simulink model "FlightControllers"  (R2021a)
settings: Solver=ode4  StartTime=0.0  StopTime=200  FixedStep=0.01  RelTol=1e-3
undefined symbols (not defined in the file): g, U0
libraries: aerolibasang x1
settings Model: Creator=User01  LastModifiedBy=User01

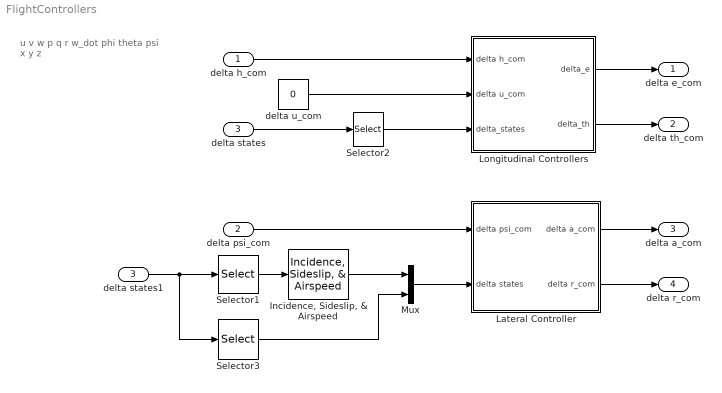
== system FlightControllers ==
  note: u
      | v
      | w
      |
      | p
      | q
      | r
      |
      | w_dot
      |
      | phi
      | theta
      | psi
      |
      | x
      | y
      | z
  delta h_com : Inport
  delta psi_com : Inport  Port=2
  delta states : Inport  Port=3
  "Incidence, Sideslip, & Airspeed" : aerolibasang/Incidence, Sideslip, & Airspeed
  Lateral Controller : Subsystem
  Longitudinal Controllers : Subsystem
  Mux : Mux  Inputs=2
  Selector1 : Selector  InputPortWidth=13  IndexOptions=Index vector (dialog)  Indices=[1:3]  OutputSizes=1
  Selector2 : Selector  InputPortWidth=13  IndexOptions=Index vector (dialog)  Indices=[1 3 5 9 13]  OutputSizes=1
  Selector3 : Selector  InputPortWidth=13  IndexOptions=Index vector (dialog)  Indices=[4 6 8 10]  OutputSizes=1
  delta states1 : InportShadow  Port=3
  delta u_com : Constant  Value=0
  delta e_com : Outport
  delta th_com : Outport  Port=2
  delta a_com : Outport  Port=3
  delta r_com : Outport  Port=4
  wires:
  Longitudinal Controllers/1(delta_e) -> delta e_com/1
  Longitudinal Controllers/2(delta_th) -> delta th_com/1
  Selector2/1 -> Longitudinal Controllers/3(delta_states)
  delta h_com/1 -> Longitudinal Controllers/1(delta h_com)
  delta states/1 -> Selector2/1
  delta u_com/1 -> Longitudinal Controllers/2(delta u_com)
  Lateral Controller/1(delta a_com) -> delta a_com/1
  Lateral Controller/2(delta r_com) -> delta r_com/1
  delta psi_com/1 -> Lateral Controller/1(delta psi_com)
  delta states1/1 -> Selector3/1, Selector1/1
  Selector1/1 -> "Incidence, Sideslip, & Airspeed"/1
  "Incidence, Sideslip, & Airspeed"/2 -> Mux/1
  Mux/1 -> Lateral Controller/2(delta states)
  Selector3/1 -> Mux/2

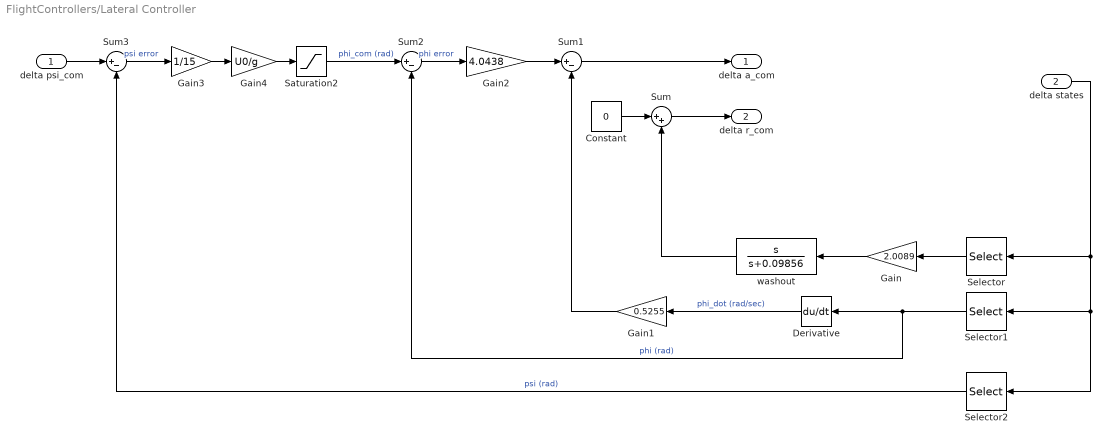
== system FlightControllers/Lateral Controller ==
  delta psi_com : Inport
  delta states : Inport  Port=2
  Constant : Constant  Value=0
  Derivative : Derivative
  Gain : Gain  Gain=2.0089
  Gain1 : Gain  Gain=0.5255
  Gain2 : Gain  Gain=4.0438
  Gain3 : Gain  Gain=1/15
  Gain4 : Gain  Gain=U0/g
  Saturation2 : Saturate  UpperLimit=30*pi/180  LowerLimit=-30*pi/180
  Selector : Selector  InputPortWidth=5  IndexOptions=Index vector (dialog)  Indices=3  OutputSizes=1
  Selector1 : Selector  InputPortWidth=5  IndexOptions=Index vector (dialog)  Indices=4  OutputSizes=1
  Selector2 : Selector  InputPortWidth=5  IndexOptions=Index vector (dialog)  Indices=5  OutputSizes=1
  Sum : Sum  Inputs=|++
  Sum1 : Sum  Inputs=|+-
  Sum2 : Sum  Inputs=|+-
  Sum3 : Sum  Inputs=|+-
  washout : TransferFcn  Numerator=[1 0]  Denominator=[1 0.09856]
  delta a_com : Outport
  delta r_com : Outport  Port=2
  wires:
  Derivative/1 -> Gain1/1  "phi_dot (rad/sec)"
  delta states/1 -> Selector2/1, Selector1/1, Selector/1
  Sum/1 -> delta r_com/1
  Sum3/1 -> Gain3/1  "psi error"
  Constant/1 -> Sum/1
  washout/1 -> Sum/2
  Gain2/1 -> Sum1/1
  Gain/1 -> washout/1
  Selector/1 -> Gain/1
  Saturation2/1 -> Sum2/1  "phi_com (rad)"
  Sum2/1 -> Gain2/1  "phi error"
  Selector2/1 -> Sum3/2  "psi (rad)"
  Gain1/1 -> Sum1/2
  Gain3/1 -> Gain4/1
  Selector1/1 -> Derivative/1, Sum2/2  "phi (rad)"
  Gain4/1 -> Saturation2/1
  delta psi_com/1 -> Sum3/1
  Sum1/1 -> delta a_com/1

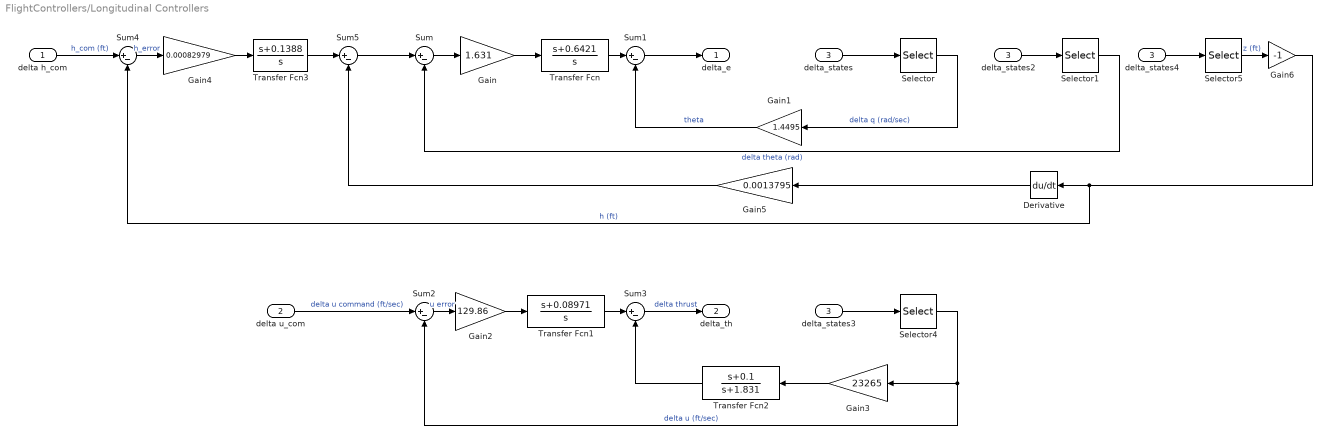
== system FlightControllers/Longitudinal Controllers ==
  delta h_com : Inport
  delta u_com : Inport  Port=2
  delta_states : Inport  Port=3
  Derivative : Derivative
  Gain : Gain  Gain=1.631
  Gain1 : Gain  Gain=1.4495
  Gain2 : Gain  Gain=129.86
  Gain3 : Gain  Gain=23265
  Gain4 : Gain  Gain=0.00082979
  Gain5 : Gain  Gain=0.0013795
  Gain6 : Gain  Gain=-1
  Selector : Selector  InputPortWidth=5  IndexOptions=Index vector (dialog)  Indices=3  OutputSizes=1
  Selector1 : Selector  InputPortWidth=5  IndexOptions=Index vector (dialog)  Indices=4  OutputSizes=1
  Selector4 : Selector  InputPortWidth=5  IndexOptions=Index vector (dialog)  Indices=1  OutputSizes=1
  Selector5 : Selector  InputPortWidth=5  IndexOptions=Index vector (dialog)  Indices=5  OutputSizes=1
  Sum{,1..5} (6 alike) : Sum  Inputs=|+-
  Transfer Fcn : TransferFcn  Numerator=[1 0.6421]  Denominator=[1 0]
  Transfer Fcn1 : TransferFcn  Numerator=[1 0.08971]  Denominator=[1 0]
  Transfer Fcn2 : TransferFcn  Numerator=[1 0.1]  Denominator=[1 1.831]
  Transfer Fcn3 : TransferFcn  Numerator=[1 0.1388]  Denominator=[1 0]
  delta_states2 : InportShadow  Port=3
  delta_states3 : InportShadow  Port=3
  delta_states4 : InportShadow  Port=3
  delta_e : Outport
  delta_th : Outport  Port=2
  wires:
  Sum1/1 -> delta_e/1
  Transfer Fcn/1 -> Sum1/1
  Gain/1 -> Transfer Fcn/1
  Gain1/1 -> Sum1/2  "theta"
  Sum/1 -> Gain/1
  delta h_com/1 -> Sum4/1  "h_com (ft)"
  delta_states/1 -> Selector/1
  Selector/1 -> Gain1/1  "delta q (rad/sec)"
  delta_states2/1 -> Selector1/1
  Selector1/1 -> Sum/2  "delta theta (rad)"
  delta_states3/1 -> Selector4/1
  delta u_com/1 -> Sum2/1  "delta u command (ft/sec)"
  Selector4/1 -> Gain3/1, Sum2/2  "delta u (ft/sec)"
  Transfer Fcn1/1 -> Sum3/1
  Sum2/1 -> Gain2/1  "u error"
  Sum3/1 -> delta_th/1  "delta thrust"
  Transfer Fcn2/1 -> Sum3/2
  Gain2/1 -> Transfer Fcn1/1
  Gain3/1 -> Transfer Fcn2/1
  delta_states4/1 -> Selector5/1
  Gain6/1 -> Derivative/1, Sum4/2  "h (ft)"
  Transfer Fcn3/1 -> Sum5/1
  Sum5/1 -> Sum/1
  Gain4/1 -> Transfer Fcn3/1
  Sum4/1 -> Gain4/1  "h_error"
  Gain5/1 -> Sum5/2
  Derivative/1 -> Gain5/1
  Selector5/1 -> Gain6/1  "z (ft)"
